simulink library "ox_lib"  (Simulink 7.5)
settings: Solver=ode45  SolverMode=SingleTasking  StartTime=0.0  StopTime=10.0  RelTol=1e-3
PostLoadFcn:
  | % Stub definitions for mask variables
  | delay_depth=16;
  | n_bits=8;
  | bin_pt=7;
libraries: xbsIndex_r4 x698, casper_library x173, ox_lib x8, xps_library x2
(part 2 of 8)

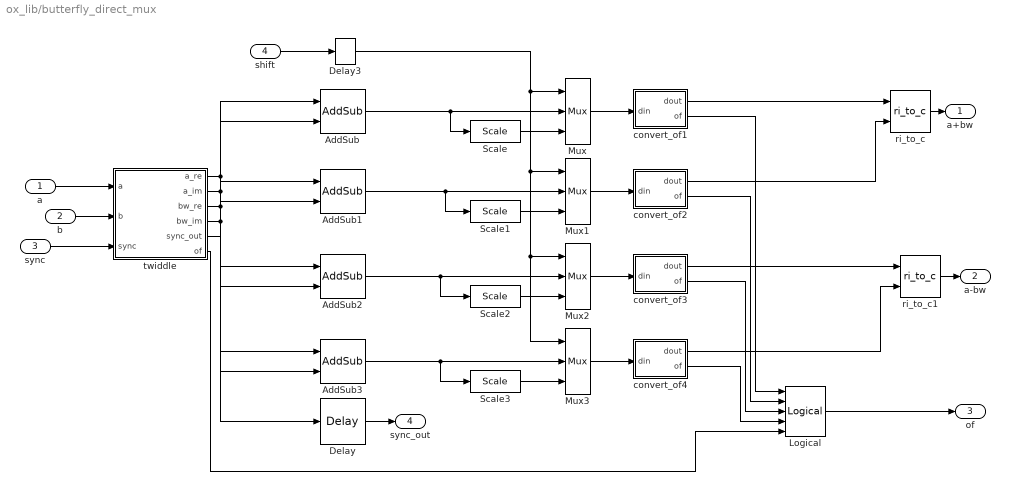
== system ox_lib/butterfly_direct_mux ==
  a : Inport  OutDataType=sfix(16)  OutScaling=2^0
  b : Inport  Port=2  OutDataType=sfix(16)  OutScaling=2^0
  sync : Inport  Port=3  OutDataType=sfix(16)  OutScaling=2^0
  shift : Inport  Port=4  OutDataType=sfix(16)  OutScaling=2^0
  AddSub : xbsIndex_r4/AddSub  mode=Addition  use_carryin=off  use_carryout=off  en=off  latency=add_latency  precision=Full  arith_type=Unsigned  n_bits=8  bin_pt=2  quantization=Truncate  overflow=Wrap  dbl_ovrd=off  use_behavioral_HDL=on  hw_selection=DSP48  pipelined=on  use_rpm=on  block_type=addsub
      settings: xl_area=[0, 0, 0, 0, 0, 0, 0]  block_version=9.1.01
  AddSub1 : xbsIndex_r4/AddSub  mode=Addition  use_carryin=off  use_carryout=off  en=off  latency=add_latency  precision=Full  arith_type=Unsigned  n_bits=8  bin_pt=2  quantization=Truncate  overflow=Wrap  dbl_ovrd=off  use_behavioral_HDL=on  hw_selection=DSP48  pipelined=on  use_rpm=on  block_type=addsub
      settings: xl_area=[0, 0, 0, 0, 0, 0, 0]  block_version=9.1.01
  AddSub2 : xbsIndex_r4/AddSub  mode=Subtraction  use_carryin=off  use_carryout=off  en=off  latency=add_latency  precision=Full  arith_type=Unsigned  n_bits=8  bin_pt=2  quantization=Truncate  overflow=Wrap  dbl_ovrd=off  use_behavioral_HDL=on  hw_selection=DSP48  pipelined=on  use_rpm=on  block_type=addsub
      settings: xl_area=[0, 0, 0, 0, 0, 0, 0]  block_version=9.1.01
  AddSub3 : xbsIndex_r4/AddSub  mode=Subtraction  use_carryin=off  use_carryout=off  en=off  latency=add_latency  precision=Full  arith_type=Unsigned  n_bits=8  bin_pt=2  quantization=Truncate  overflow=Wrap  dbl_ovrd=off  use_behavioral_HDL=on  hw_selection=DSP48  pipelined=on  use_rpm=on  block_type=addsub
      settings: xl_area=[0, 0, 0, 0, 0, 0, 0]  block_version=9.1.01
  Delay : xbsIndex_r4/Delay  en=off  latency=add_latency + 2  dbl_ovrd=off  reg_retiming=off  block_type=delay
      settings: xl_area=[0, 0, 0, 0, 0, 0, 0]  block_version=9.1.01
  Delay3 : xbsIndex_r4/Delay  en=off  latency=add_latency  dbl_ovrd=off  reg_retiming=off  block_type=delay
      settings: xl_area=[0, 0, 0, 0, 0, 0, 0]  block_version=9.1.01
  Logical : xbsIndex_r4/Logical  logical_function=OR  inputs=5  en=off  latency=0  precision=Full  arith_type=Unsigned  n_bits=16  bin_pt=0  align_bp=on  dbl_ovrd=off  block_type=logical
      settings: block_version=10.1.1
  Mux{,1..3} (4 alike) : xbsIndex_r4/Mux  inputs=2  en=off  latency=1  precision=Full  arith_type="Signed  (2's comp)"  n_bits=8  bin_pt=2  quantization=Truncate  overflow=Wrap  dbl_ovrd=off  block_type=mux
      settings: xl_area=[0, 0, 0, 0, 0, 0, 0]  block_version=9.1.01
  Scale{,1..3} (4 alike) : xbsIndex_r4/Scale  scale_factor=-1  dbl_ovrd=off  block_type=scale
      settings: infoedit=Scales input by a power of two by adjusting the binary point position.<P><P>Hardware notes: In hardware this block costs nothing.  block_version=9.1.01
  convert_of1 : Subsystem  AncestorBlock=casper_library/Misc/convert_of  mask(convert_of){bit_width_i=20, binary_point_i=18, bit_width_o=18, binary_point_o=17, latency=1, overflow=Wrap, quantization=Truncate}
      mask prompts: bit_width_i "Bit Width In"; binary_point_i "Binary Point In"; bit_width_o "Bit Width Out"; binary_point_o "Binary Point Out"; overflow "Overflow Behaviour"; quantization "Quantization Behaviour"
      mask help:
      | Converts from one 2's complement bit-width
      | and/or binary point position to another.
      | Includes underflow/overflow indicator.
      mask init:
      | convert_of_init(gcb, ...
      |     'bit_width_i', bit_width_i, ...
      |     'binary_point_i', binary_point_i, ...
      |     'bit_width_o', bit_width_o, ...
      |     'binary_point_o', binary_point_o, ...
      |     'latency', latency, ...
      |     'overflow', overflow, ...
      |     'quantization', quantization);
      settings: AttributesFormatString=[20,18]->[18,17]
      mask StyleString: edit,edit,edit,edit,edit,popup(Wrap|Saturate|Error),popup(Truncate|Round  (unbiased: +/- Inf)|Round  (unbiased: even values))
  convert_of2 : Subsystem  AncestorBlock=casper_library/FFTs/butterfly_direct/convert_of1  mask(convert_of){bit_width_i=20, binary_point_i=18, bit_width_o=18, binary_point_o=17, latency=1, overflow=Wrap, quantization=Truncate}
      mask prompts: bit_width_i "Bit Width In"; binary_point_i "Binary Point In"; bit_width_o "Bit Width Out"; binary_point_o "Binary Point Out"; overflow "Overflow Behaviour"; quantization "Quantization Behaviour"
      mask help:
      | Converts from one 2's complement bit-width
      | and/or binary point position to another.
      | Includes underflow/overflow indicator.
      mask init: same as ox_lib/butterfly_direct_mux/convert_of1
      settings: AttributesFormatString=[20,18]->[18,17]
      mask StyleString: edit,edit,edit,edit,edit,popup(Wrap|Saturate|Error),popup(Truncate|Round  (unbiased: +/- Inf)|Round  (unbiased: even values))
  convert_of3 : Subsystem  AncestorBlock=casper_library/FFTs/butterfly_direct/convert_of1  mask(convert_of){bit_width_i=20, binary_point_i=18, bit_width_o=18, binary_point_o=17, latency=1, overflow=Wrap, quantization=Truncate}
      mask prompts: bit_width_i "Bit Width In"; binary_point_i "Binary Point In"; bit_width_o "Bit Width Out"; binary_point_o "Binary Point Out"; overflow "Overflow Behaviour"; quantization "Quantization Behaviour"
      mask help:
      | Converts from one 2's complement bit-width
      | and/or binary point position to another.
      | Includes underflow/overflow indicator.
      mask init: same as ox_lib/butterfly_direct_mux/convert_of1
      settings: AttributesFormatString=[20,18]->[18,17]
      mask StyleString: edit,edit,edit,edit,edit,popup(Wrap|Saturate|Error),popup(Truncate|Round  (unbiased: +/- Inf)|Round  (unbiased: even values))
  convert_of4 : Subsystem  AncestorBlock=casper_library/FFTs/butterfly_direct/convert_of1  mask(convert_of){bit_width_i=20, binary_point_i=18, bit_width_o=18, binary_point_o=17, latency=1, overflow=Wrap, quantization=Truncate}
      mask prompts: bit_width_i "Bit Width In"; binary_point_i "Binary Point In"; bit_width_o "Bit Width Out"; binary_point_o "Binary Point Out"; overflow "Overflow Behaviour"; quantization "Quantization Behaviour"
      mask help:
      | Converts from one 2's complement bit-width
      | and/or binary point position to another.
      | Includes underflow/overflow indicator.
      mask init: same as ox_lib/butterfly_direct_mux/convert_of1
      settings: AttributesFormatString=[20,18]->[18,17]
      mask StyleString: edit,edit,edit,edit,edit,popup(Wrap|Saturate|Error),popup(Truncate|Round  (unbiased: +/- Inf)|Round  (unbiased: even values))
  ri_to_c : casper_library/Misc/ri_to_c  SystemSampleTime=-1
  ri_to_c1 : casper_library/Misc/ri_to_c  SystemSampleTime=-1
  twiddle : Subsystem  AncestorBlock=ox_lib/Twiddle/twiddle_pass_through  mask(twiddle_pass_through){input_bit_width=18, coeff_bit_width=18, add_latency=1, mult_latency=3, bram_latency=3, use_hdl=on, use_embedded=off, quantization=Truncate, overflow=Wrap, mux_factor=0}
      mask prompts: input_bit_width "Input Bit Width"; coeff_bit_width "Coefficient Bit Width"; add_latency "Add Latency"; mult_latency "Mult Latency"; bram_latency "BRAM Latency"; use_hdl "Use behavioural HDL for multipliers"; use_embedded "Use embedded multipliers"; quantization "Quantization Behavior"; overflow "Overflow Behavior"; mux_factor "Multiplex factor (2^?)"
      mask help:
      | Used in FFT library. Used when coefficients
      | are 2^0 i.e just pass data through without delays
      mask StyleString: edit,edit,edit,edit,edit,checkbox,checkbox,popup(Truncate|Round  (unbiased: +/- Inf)|Round  (unbiased: Even Values)),popup(Wrap|Saturate|Error),edit
  a+bw : Outport  OutDataType=sfix(16)  OutScaling=2^0
  a-bw : Outport  Port=2  OutDataType=sfix(16)  OutScaling=2^0
  of : Outport  Port=3  OutDataType=sfix(16)  OutScaling=2^0
  sync_out : Outport  Port=4  OutDataType=sfix(16)  OutScaling=2^0
  wires:
  Logical/1 -> of/1
  Delay3/1 -> Mux/1, Mux1/1, Mux2/1, Mux3/1
  Scale/1 -> Mux/3
  shift/1 -> Delay3/1
  AddSub/1 -> Scale/1, Mux/2
  Delay/1 -> sync_out/1
  ri_to_c1/1 -> a-bw/1
  ri_to_c/1 -> a+bw/1
  a/1 -> twiddle/1(a)
  b/1 -> twiddle/2(b)
  sync/1 -> twiddle/3(sync)
  twiddle/1(a_re) -> AddSub/1, AddSub2/1
  twiddle/2(a_im) -> AddSub1/1, AddSub3/1
  twiddle/3(bw_re) -> AddSub/2, AddSub2/2
  twiddle/4(bw_im) -> AddSub1/2, AddSub3/2
  twiddle/5(sync_out) -> Delay/1
  Mux/1 -> convert_of1/1(din)
  convert_of1/1(dout) -> ri_to_c/1
  Scale1/1 -> Mux1/3
  AddSub1/1 -> Mux1/2, Scale1/1
  Mux1/1 -> convert_of2/1(din)
  convert_of2/1(dout) -> ri_to_c/2
  Scale2/1 -> Mux2/3
  AddSub2/1 -> Mux2/2, Scale2/1
  Mux2/1 -> convert_of3/1(din)
  convert_of3/1(dout) -> ri_to_c1/1
  Scale3/1 -> Mux3/3
  AddSub3/1 -> Mux3/2, Scale3/1
  Mux3/1 -> convert_of4/1(din)
  convert_of4/1(dout) -> ri_to_c1/2
  convert_of1/2(of) -> Logical/1
  convert_of2/2(of) -> Logical/2
  convert_of3/2(of) -> Logical/3
  convert_of4/2(of) -> Logical/4
  twiddle/6(of) -> Logical/5

== system ox_lib/cplx_truncate ==
  in : Inport  OutDataType=sfix(16)  OutScaling=2^0
  c_to_ri : casper_library/Misc/c_to_ri  SystemSampleTime=-1  n_bits=in_bits  bin_pt=in_bits-1
      settings: AttributesFormatString=19_18 r/i
  convert_im : xbsIndex_r4/Convert  arith_type="Signed  (2's comp)"  n_bits=out_bits  bin_pt=out_bits-1  quantization=Truncate  overflow=Wrap  latency=0  dbl_ovrd=off  pipeline=on  block_type=convert
      settings: xl_area=[0, 0, 0, 0, 0, 0, 0]  block_version=10.1.3
  convert_re : xbsIndex_r4/Convert  arith_type="Signed  (2's comp)"  n_bits=out_bits  bin_pt=out_bits-1  quantization=Truncate  overflow=Wrap  latency=0  dbl_ovrd=off  pipeline=on  block_type=convert
      settings: xl_area=[0, 0, 0, 0, 0, 0, 0]  block_version=10.1.3
  ri_to_c : casper_library/Misc/ri_to_c  SystemSampleTime=-1
  out : Outport  OutDataType=sfix(16)  OutScaling=2^0
  wires:
  convert_im/1 -> ri_to_c/2
  c_to_ri/2 -> convert_im/1
  in/1 -> c_to_ri/1
  ri_to_c/1 -> out/1
  convert_re/1 -> ri_to_c/1
  c_to_ri/1 -> convert_re/1

== system ox_lib/fft_biplex_mux ==
  pol1 : Inport  OutDataType=sfix(16)  OutScaling=2^0
  pol2 : Inport  Port=2  OutDataType=sfix(16)  OutScaling=2^0
  sync : Inport  Port=3  OutDataType=sfix(16)  OutScaling=2^0
  shift : Inport  Port=4  OutDataType=sfix(16)  OutScaling=2^0
  biplex_core_mux : ox_lib/biplex_core_mux  SystemSampleTime=-1  FFTSize=FFTSize  input_bit_width=18  coeff_bit_width=18  quantization=Truncate  overflow=Wrap  add_latency=1  mult_latency=2  bram_latency=3  arch=Virtex2Pro  opt_target=Multipliers  coeffs_bit_limit=8  delays_bit_limit=8  specify_mult=off  mult_spec="[2                                      2                                      2]"  dsp48_adders=off  mux_factor=0
      settings: AttributesFormatString=|
      | FFTSize=3,
      |  opt_target=Multipliers,
      |  arch=Virtex2Pro
  biplex_cplx_unscrambler : Subsystem  mask{FFTSize=4, bram_latency=3}
      mask prompts: FFTSize "Size of FFT: (2^? pnts)"; bram_latency "BRAM Latency"
      mask init:
      | blk = gcb;
      | if same_state(blk, 'FFTSize', FFTSize, 'bram_latency', bram_latency), return, end
      | map = bit_reverse(0:2^(FFTSize-1)-1, FFTSize-1);
      | set_param([blk,'/reorder'],'map',mat2str([map,map+2^(FFTSize-1)]));
      | set_param([blk,'/reorder'],'bram_latency', num2str(bram_latency));
      | set_param([blk,'/reorder1'],'map',mat2str([map+2^(FFTSize-1),map]));
      | set_param([blk,'/reorder1'],'bram_latency', num2str(bram_latency));
      | save_state(blk, 'FFTSize', FFTSize, 'bram_latency', bram_latency);
  pol1_out : Outport  OutDataType=sfix(16)  OutScaling=2^0
  pol2_out : Outport  Port=2  OutDataType=sfix(16)  OutScaling=2^0
  of : Outport  Port=3  OutDataType=sfix(16)  OutScaling=2^0
  sync_out : Outport  Port=4  OutDataType=sfix(16)  OutScaling=2^0
  wires:
  biplex_core_mux/3 -> of/1
  biplex_cplx_unscrambler/1(pol1) -> pol1_out/1
  shift/1 -> biplex_core_mux/4
  sync/1 -> biplex_core_mux/3
  pol2/1 -> biplex_core_mux/2
  pol1/1 -> biplex_core_mux/1
  biplex_core_mux/1 -> biplex_cplx_unscrambler/1(even)
  biplex_core_mux/2 -> biplex_cplx_unscrambler/2(odd)
  biplex_core_mux/4 -> biplex_cplx_unscrambler/3(sync)
  biplex_cplx_unscrambler/2(pol2) -> pol2_out/1
  biplex_cplx_unscrambler/3(sync_out) -> sync_out/1

== system ox_lib/fft_mux ==
  sync : Inport  OutDataType=sfix(16)  OutScaling=2^0
  shift : Inport  Port=2  OutDataType=sfix(16)  OutScaling=2^0
  pol0 : Inport  Port=3
  pol1 : Inport  Port=4
  fft_biplex0 : Subsystem  AncestorBlock=ox_lib/fft_biplex_mux  mask(fft_biplex_mux){FFTSize=4, mux_factor=0, input_bit_width=18, coeff_bit_width=18, quantization=Truncate, overflow=Wrap, add_latency=1, mult_latency=3, bram_latency=3, arch=Virtex2Pro, opt_target=Multipliers, coeffs_bit_limit=8, delays_bit_limit=9, specify_mult=off, mult_spec=getfield( getfield( get_param( gcb,'UserData' ), 'parameters'),'mult_spec'), dsp48_adders=off}
      mask prompts: FFTSize "Size of FFT: (2^? pnts)"; mux_factor "Multiplexing factor (2^?)"; input_bit_width "Input/Output Bit Width"; coeff_bit_width "Coefficient Bit Width"; quantization "Quantization Behavior"; overflow "Overflow Behavior"; add_latency "Add Latency"; mult_latency "Mult Latency"; bram_latency "BRAM Latency"; arch "Architecture"; opt_target "Optimisation Target"; coeffs_bit_limit "Number bits above which to store stage's coefficients in BRAM (2^? bits)"; delays_bit_limit "Number bits above which to implent stage's delays in BRAM (2^? bits)"; specify_mult "Specify multiplier use (behavioral HDL if not specified)"; mult_spec "Multiplier specification (0=core, 1=embedded, 2=behavioural) (left=1st stage)"; dsp48_adders "Use DSP48s for adders"
      mask init: same as ox_lib/fft_biplex_mux
      settings: AttributesFormatString=|
      | FFTSize=4,
      |  arch=Virtex2Pro,
      |  opt_target=Multipliers
      mask StyleString: edit,edit,edit,edit,popup(Truncate|Round  (unbiased: +/- Inf)|Round  (unbiased: Even Values)),popup(Wrap|Saturate|Error),edit,edit,edit,popup(Virtex2Pro|Virtex5),popup(Logic|Multipliers),edit,edit,checkbox,edit,checkbox
      mask CallbackString:
      | % fft_size = eval(get_param(gcb, 'FFTSize'));
      | % old_vec = eval(get_param(gcb, 'mult_spec'));
      | 
      | % vec = 2.*ones(1,fft_size);
      | % old_size = length(old_vec);
      | 
      | % if(old_size <= fft_size),
      | %    size = old_size;
      | % else,
      | %     size = fft_size;
      | % end
      | 
      | % for n = 1:size, vec(n) = old_vec(n); end
      | % set_param(gcb, 'mult_spec', mat2str(vec));|||||||||||||specify_mult = get_param(gcb,'specify_mult');
      | visibs = get_param(gcb, 'MaskVisibilities');
      | 
      | if( strcmp(specify_mult,'off')), visibs{14} = 'off';
      | else, visibs{14} = 'on';
      | end
      | set_param(gcb, 'MaskVisibilities', visibs);
      | |% vec = eval( get_param(gcb, 'mult_spec'));
      | % vec_size = length(vec);
      | % fft_size = eval( get_param(gcb, 'FFTSize'));
      | % new_vec = 2.*ones(1, fft_size);
      | 
      | % if(vec_size <= fft_size), size = vec_size;
      | % else size = fft_size;
      | % end
      | 
      | % for n=1:size
      | %     new_vec(n) = vec(n);
      | % end
      | % set_param(gcb, 'mult_spec', mat2str(new_vec));|
  sync_out : Outport
  out0 : Outport  Port=2
  out1 : Outport  Port=3
  of : Outport  Port=4
  wires:
  pol0/1 -> fft_biplex0/1(pol1)
  pol1/1 -> fft_biplex0/2(pol2)
  shift/1 -> fft_biplex0/4(shift)
  sync/1 -> fft_biplex0/3(sync)
  fft_biplex0/1(pol1_out) -> out0/1
  fft_biplex0/2(pol2_out) -> out1/1
  fft_biplex0/4(sync_out) -> sync_out/1
  fft_biplex0/3(of) -> of/1

== system ox_lib/fft_stage_n_mux ==
  in1 : Inport  OutDataType=sfix(16)  OutScaling=2^0
  in2 : Inport  Port=2  OutDataType=sfix(16)  OutScaling=2^0
  of_in : Inport  Port=3  OutDataType=sfix(16)  OutScaling=2^0
  sync : Inport  Port=4  OutDataType=sfix(16)  OutScaling=2^0
  shift : Inport  Port=5  OutDataType=sfix(16)  OutScaling=2^0
  Counter : xbsIndex_r4/Counter  cnt_type=Free Running  cnt_to=Inf  operation=Up  start_count=0  cnt_by_val=1  arith_type=Unsigned  n_bits=FFTSize-FFTStage+1+mux_factor  bin_pt=0  load_pin=off  rst=on  en=off  explicit_period=off  period=1  dbl_ovrd=off  use_behavioral_HDL=off  implementation=Fabric  use_rpm=off  block_type=counter
      settings: xl_area=[0, 0, 0, 0, 0, 0, 0]  block_version=9.1.01
  Delay : xbsIndex_r4/Delay  en=off  latency=1  dbl_ovrd=off  reg_retiming=off  block_type=delay
      settings: xl_area=[0, 0, 0, 0, 0, 0, 0]  block_version=9.1.01
  Logical1 : xbsIndex_r4/Logical  logical_function=OR  inputs=2  en=off  latency=1  precision=Full  arith_type=Unsigned  n_bits=8  bin_pt=2  align_bp=on  dbl_ovrd=off  block_type=logical
      settings: xl_area=[0, 0, 0, 0, 0, 0, 0]  block_version=9.1.01
  Mux : xbsIndex_r4/Mux  inputs=2  en=off  latency=1  precision=Full  arith_type="Signed  (2's comp)"  n_bits=8  bin_pt=2  quantization=Truncate  overflow=Wrap  dbl_ovrd=off  block_type=mux
      settings: xl_area=[0, 0, 0, 0, 0, 0, 0]  block_version=9.1.01
  Mux1 : xbsIndex_r4/Mux  inputs=2  en=off  latency=1  precision=Full  arith_type="Signed  (2's comp)"  n_bits=8  bin_pt=2  quantization=Truncate  overflow=Wrap  dbl_ovrd=off  block_type=mux
      settings: xl_area=[0, 0, 0, 0, 0, 0, 0]  block_version=9.1.01
  Slice : xbsIndex_r4/Slice  nbits=1  boolean_output=on  mode=Lower Bit Location + Width  bit1=-(FFTStage - 1)  base1=MSB of Input  bit0=FFTStage - 1  base0=LSB of Input  dbl_ovrd=off  block_type=slice
      settings: infoedit="Extracts a given range of bits from each input sample and presents it at the output.  The output type is ordinarily unsigned with binary point at zero, but can be Boolean when the slice is one bit wide.<P><P>Hardware notes: In hardware this block costs nothing."  block_version=9.1.01
  Slice1 : xbsIndex_r4/Slice  nbits=1  boolean_output=off  mode=Upper Bit Location + Width  bit1=0  base1=MSB of Input  bit0=0  base0=LSB of Input  dbl_ovrd=off  block_type=slice
      settings: infoedit="Extracts a given range of bits from each input sample and presents it at the output.  The output type is ordinarily unsigned with binary point at zero, but can be Boolean when the slice is one bit wide.<P><P>Hardware notes: In hardware this block costs nothing."  block_version=9.1.01
  butterfly_direct_mux : ox_lib/butterfly_direct_mux  SystemSampleTime=-1  biplex=on  FFTSize=4  Coeffs=0  coeff_bit_width=18  StepPeriod=3  bram_latency=3  coeffs_bram=off  input_bit_width=18  add_latency=1  mult_latency=3  quantization=Truncate  overflow=Wrap  arch=Virtex2Pro  opt_target=Multipliers  use_hdl=on  use_embedded=off  dsp48_adders=off  mux_factor=0
      settings: AttributesFormatString=FFTSize=4, coeff_bit_width=18
  delay_b : Subsystem  AncestorBlock=casper_library/Delays/delay_slr  mask(delay_slr){DelayLen=2^(FFTSize-FFTStage+mux_factor)}
      mask prompts: DelayLen "Delay by:"
      mask help: A delay block that uses slices (SLR16s) for its storage.
      mask Help: eval('xlWeb(''http://casper.berkeley.edu/wiki/Delay_slr'')')
  delay_f : Subsystem  AncestorBlock=casper_library/Delays/delay_slr  mask(delay_slr){DelayLen=2^(FFTSize-FFTStage+mux_factor)}
      mask prompts: DelayLen "Delay by:"
      mask help: A delay block that uses slices (SLR16s) for its storage.
      mask Help: eval('xlWeb(''http://casper.berkeley.edu/wiki/Delay_slr'')')
  sync_delay : casper_library/Delays/sync_delay  SystemSampleTime=-1  DelayLen=2^(FFTSize - FFTStage+mux_factor)
  out1 : Outport  OutDataType=sfix(16)  OutScaling=2^0
  out2 : Outport  Port=2  OutDataType=sfix(16)  OutScaling=2^0
  of : Outport  Port=3  OutDataType=sfix(16)  OutScaling=2^0
  sync_out : Outport  Port=4  OutDataType=sfix(16)  OutScaling=2^0
  wires:
  shift/1 -> Slice/1
  of_in/1 -> Logical1/2
  Logical1/1 -> of/1
  Delay/1 -> sync_delay/1
  sync/1 -> Counter/1, Delay/1
  Counter/1 -> Slice1/1
  Mux/1 -> butterfly_direct_mux/2
  Mux1/1 -> delay_b/1(In1)
  delay_f/1(Out1) -> Mux1/3, Mux/2
  in1/1 -> Mux/3, Mux1/2
  Slice1/1 -> Mux/1, Mux1/1
  in2/1 -> delay_f/1(In1)
  delay_b/1(Out1) -> butterfly_direct_mux/1
  sync_delay/1 -> butterfly_direct_mux/3
  Slice/1 -> butterfly_direct_mux/4
  butterfly_direct_mux/3 -> Logical1/1
  butterfly_direct_mux/2 -> out2/1
  butterfly_direct_mux/1 -> out1/1
  butterfly_direct_mux/4 -> sync_out/1

== system ox_lib/global_slave_reg ==
  sim_val : Inport
  Register : xbsIndex_r4/Register  init=0  rst=off  en=on  dbl_ovrd=off  block_type=register
      settings: block_version=11.4
  Simulation Multiplexer : xbsIndex_r4/Simulation Multiplexer  sim_sel=1  hw_sel=2  block_type=simmux
      settings: infoedit="Distinguish input subsystems as \"simulation only\" and \"generation only\".  The input specified For Simulation will be used during Simulink simulation.  The input specified For Generation will be used during code generation.  This block will typically be used on the output of a HW Co-Simulation, Black Box, or ModelSim subsystem.<br><br>Hardware Notes: This block costs nothing."  block_version=11.4
  data_width : xbsIndex_r4/Slice  nbits=data_width  boolean_output=off  mode=Lower Bit Location + Width  bit1=0  base1=MSB of Input  bit0=0  base0=LSB of Input  dbl_ovrd=off  block_type=slice
  data_width1 : xbsIndex_r4/Slice  nbits=data_width  boolean_output=off  mode=Lower Bit Location + Width  bit1=0  base1=MSB of Input  bit0=0  base0=LSB of Input  dbl_ovrd=off  block_type=slice
  en_sel : xbsIndex_r4/Slice  nbits=1  boolean_output=on  mode=Lower Bit Location + Width  bit1=0  base1=MSB of Input  bit0=enable_bit  base0=LSB of Input  dbl_ovrd=off  block_type=slice
  pipeline1 : casper_library/Delays/pipeline  SystemSampleTime=-1  latency=latency
  pipeline2 : casper_library/Delays/pipeline  SystemSampleTime=-1  latency=latency
  simulation_val : xbsIndex_r4/Gateway In  arith_type="Signed  (2's comp)"  n_bits=16  bin_pt=14  quantization="Round  (unbiased: +/- Inf)"  overflow=Saturate  period=1  dbl_ovrd=off  timing_constraint=None  locs_specified=off  LOCs={}  hdl_port=on  block_type=gatewayin
      settings: infoedit="Gateway in block.  Converts inputs of type Simulink integer, double and fixed point to  Xilinx fixed point type.<br><br>Hardware notes:  In hardware these blocks become top level input ports."  block_version=11.4
  dout : Outport
  wires:
  data_width1/1 -> Simulation Multiplexer/1
  Simulation Multiplexer/1 -> dout/1
  sim_val/1 -> simulation_val/1
  data_width/1 -> Register/1
  en_sel/1 -> Register/2
  Register/1 -> Simulation Multiplexer/2
  simulation_val/1 -> data_width1/1
  [reg_addr] -> pipeline2/1
  [reg_data] -> pipeline1/1
  pipeline2/1 -> en_sel/1
  pipeline1/1 -> data_width/1

== system ox_lib/global_sw_ctrl ==
  err_clear_sim10 : Constant  Value=0  OutDataType=sfix(16)  OutScaling=2^0
  err_clear_sim5 : Constant  Value=0  OutDataType=sfix(16)  OutScaling=2^0
  reg_addr : xps_library/software register  Tag=xps:sw_reg  SystemSampleTime=-1  io_dir=From Processor  arith_type=Unsigned  bitwidth=32  bin_pt=0  sample_period=1  gw_name=ox_lib_global_sw_ctrl_reg_addr_user_data_out
      link override b_2x_8a_r310b_base_ant0_user_data_out: arith_type=Unsigned  n_bits=32  bin_pt=0  period=1
      link override r_2x_8a_r310b_base_ant0_user_data_out: arith_type=Unsigned  n_bits=32  bin_pt=0  period=1
      link override r_2x_8a_r311a_base_ant0_user_data_out: arith_type=Unsigned  n_bits=32  bin_pt=0  period=1
      link override r_2x_8a_r311b_1_base_ant0_user_data_out: arith_type=Unsigned  n_bits=32  bin_pt=0  period=1
      link override r_2x_8a_r311b_base_ant0_user_data_out: arith_type=Unsigned  n_bits=32  bin_pt=0  period=1
      link override r_2x_8a_r320a_1_base_ant0_user_data_out: arith_type=Unsigned  n_bits=32  bin_pt=0  period=1
      link override r_2x_8a_r320b_1_base_ant0_user_data_out: arith_type=Unsigned  n_bits=32  bin_pt=0  period=1
      link override r_2x_8a_r320b_base_ant0_user_data_out: arith_type=Unsigned  n_bits=32  bin_pt=0  period=1
      link override r_4f_1x_16a_r322h_base_ant0_user_data_out: arith_type=Unsigned  n_bits=32  bin_pt=0  period=1
      link override r_4f_1x_16a_r322i_base_ant0_user_data_out: arith_type=Unsigned  n_bits=32  bin_pt=0  period=1
      link override r_4f_1x_16a_r322j_base_ant0_user_data_out: arith_type=Unsigned  n_bits=32  bin_pt=0  period=1
      link override r_4f_1x_16a_r322k_base_ant0_user_data_out: arith_type=Unsigned  n_bits=32  bin_pt=0  period=1
      link override r_4f_1x_16a_r322l_base_ant0_user_data_out: arith_type=Unsigned  n_bits=32  bin_pt=0  period=1
      link override r_4f_1x_16a_r322m_base_ant0_user_data_out: arith_type=Unsigned  n_bits=32  bin_pt=0  period=1
      link override r_4f_2x_16a_r320b_base_ant0_user_data_out: arith_type=Unsigned  n_bits=32  bin_pt=0  period=1
      link override r_4f_2x_16a_r321a_base_ant0_user_data_out: arith_type=Unsigned  n_bits=32  bin_pt=0  period=1
      link override r_4f_2x_16a_r322a_base_ant0_user_data_out: arith_type=Unsigned  n_bits=32  bin_pt=0  period=1
      link override r_4f_2x_16a_r322b_base_ant0_user_data_out: arith_type=Unsigned  n_bits=32  bin_pt=0  period=1
      link override r_4f_2x_16a_r322c_base_ant0_user_data_out: arith_type=Unsigned  n_bits=32  bin_pt=0  period=1
      link override r_4f_2x_16a_r322d_base_ant0_user_data_out: arith_type=Unsigned  n_bits=32  bin_pt=0  period=1
      link override r_4f_2x_16a_r322e_base_ant0_user_data_out: arith_type=Unsigned  n_bits=32  bin_pt=0  period=1
      link override r_4f_2x_16a_r322f_base_ant0_user_data_out: arith_type=Unsigned  n_bits=32  bin_pt=0  period=1
      link override r_4f_2x_16a_r322g_base_ant0_user_data_out: arith_type=Unsigned  n_bits=32  bin_pt=0  period=1
      link override r_4f_2x_16a_r322h_base_ant0_user_data_out: arith_type=Unsigned  n_bits=32  bin_pt=0  period=1
      link override r_4f_2x_16a_r322m_base_ant0_user_data_out: arith_type=Unsigned  n_bits=32  bin_pt=0  period=1
      link override r_4f_2x_16a_r323a_base_ant0_user_data_out: arith_type=Unsigned  n_bits=32  bin_pt=0  period=1
      link override r_r311b_xaui_test_base_ant0_user_data_out: arith_type=Unsigned  n_bits=32  bin_pt=0  period=1
  reg_data : xps_library/software register  Tag=xps:sw_reg  SystemSampleTime=-1  io_dir=From Processor  arith_type=Unsigned  bitwidth=32  bin_pt=0  sample_period=1  gw_name=ox_lib_global_sw_ctrl_reg_data_user_data_out
      link override b_2x_8a_r310b_base_ant0_user_data_out: arith_type=Unsigned  n_bits=32  bin_pt=0  period=1
      link override r_2x_8a_r310b_base_ant0_user_data_out: arith_type=Unsigned  n_bits=32  bin_pt=0  period=1
      link override r_2x_8a_r311a_base_ant0_user_data_out: arith_type=Unsigned  n_bits=32  bin_pt=0  period=1
      link override r_2x_8a_r311b_1_base_ant0_user_data_out: arith_type=Unsigned  n_bits=32  bin_pt=0  period=1
      link override r_2x_8a_r311b_base_ant0_user_data_out: arith_type=Unsigned  n_bits=32  bin_pt=0  period=1
      link override r_2x_8a_r320a_1_base_ant0_user_data_out: arith_type=Unsigned  n_bits=32  bin_pt=0  period=1
      link override r_2x_8a_r320b_1_base_ant0_user_data_out: arith_type=Unsigned  n_bits=32  bin_pt=0  period=1
      link override r_2x_8a_r320b_base_ant0_user_data_out: arith_type=Unsigned  n_bits=32  bin_pt=0  period=1
      link override r_4f_1x_16a_r322h_base_ant0_user_data_out: arith_type=Unsigned  n_bits=32  bin_pt=0  period=1
      link override r_4f_1x_16a_r322i_base_ant0_user_data_out: arith_type=Unsigned  n_bits=32  bin_pt=0  period=1
      link override r_4f_1x_16a_r322j_base_ant0_user_data_out: arith_type=Unsigned  n_bits=32  bin_pt=0  period=1
      link override r_4f_1x_16a_r322k_base_ant0_user_data_out: arith_type=Unsigned  n_bits=32  bin_pt=0  period=1
      link override r_4f_1x_16a_r322l_base_ant0_user_data_out: arith_type=Unsigned  n_bits=32  bin_pt=0  period=1
      link override r_4f_1x_16a_r322m_base_ant0_user_data_out: arith_type=Unsigned  n_bits=32  bin_pt=0  period=1
      link override r_4f_2x_16a_r320b_base_ant0_user_data_out: arith_type=Unsigned  n_bits=32  bin_pt=0  period=1
      link override r_4f_2x_16a_r321a_base_ant0_user_data_out: arith_type=Unsigned  n_bits=32  bin_pt=0  period=1
      link override r_4f_2x_16a_r322a_base_ant0_user_data_out: arith_type=Unsigned  n_bits=32  bin_pt=0  period=1
      link override r_4f_2x_16a_r322b_base_ant0_user_data_out: arith_type=Unsigned  n_bits=32  bin_pt=0  period=1
      link override r_4f_2x_16a_r322c_base_ant0_user_data_out: arith_type=Unsigned  n_bits=32  bin_pt=0  period=1
      link override r_4f_2x_16a_r322d_base_ant0_user_data_out: arith_type=Unsigned  n_bits=32  bin_pt=0  period=1
      link override r_4f_2x_16a_r322e_base_ant0_user_data_out: arith_type=Unsigned  n_bits=32  bin_pt=0  period=1
      link override r_4f_2x_16a_r322f_base_ant0_user_data_out: arith_type=Unsigned  n_bits=32  bin_pt=0  period=1
      link override r_4f_2x_16a_r322g_base_ant0_user_data_out: arith_type=Unsigned  n_bits=32  bin_pt=0  period=1
      link override r_4f_2x_16a_r322h_base_ant0_user_data_out: arith_type=Unsigned  n_bits=32  bin_pt=0  period=1
      link override r_4f_2x_16a_r322m_base_ant0_user_data_out: arith_type=Unsigned  n_bits=32  bin_pt=0  period=1
      link override r_4f_2x_16a_r323a_base_ant0_user_data_out: arith_type=Unsigned  n_bits=32  bin_pt=0  period=1
      link override r_r311b_xaui_test_base_ant0_user_data_out: arith_type=Unsigned  n_bits=32  bin_pt=0  period=1
  tag scope: reg_addr=global, reg_data=global
  wires:
  err_clear_sim5/1 -> reg_addr/1
  reg_addr/1 -> [reg_addr]
  err_clear_sim10/1 -> reg_data/1
  reg_data/1 -> [reg_data]
